simulink model "Compare_lin_nonlin"  (R2019b)
settings: Solver=FixedStepAuto  StartTime=0.0  StopTime=10  FixedStep=0.01  RelTol=1e-3
settings Model: Creator=cambr  LastModifiedBy=cambr

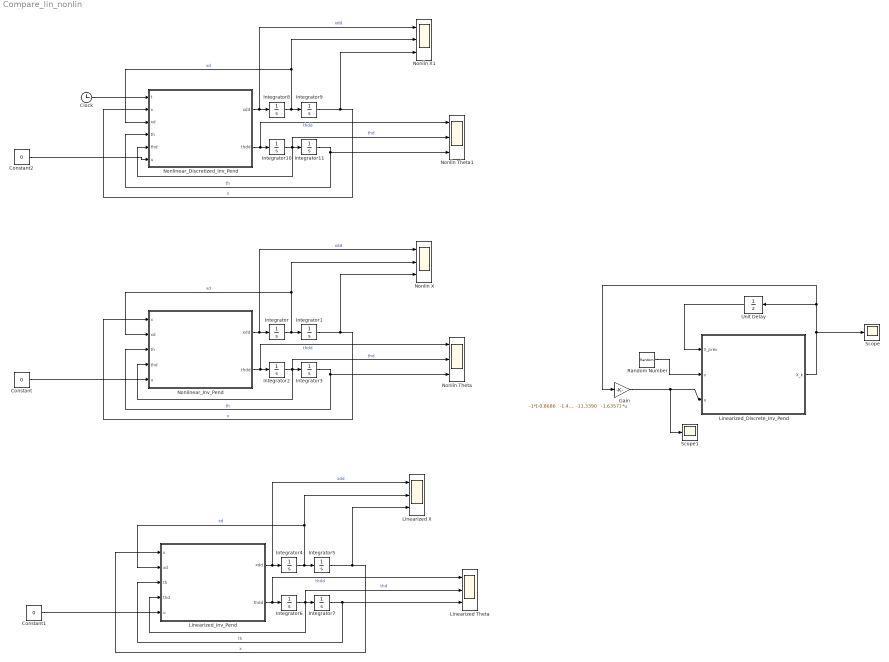
== system Compare_lin_nonlin ==
  Clock : Clock
  Constant : Constant  Value=0
  Constant1 : Constant  Value=0
  Constant2 : Constant  Value=0
  Gain : Gain  Gain="-1*[-0.8686   -1.4350  -11.3390   -1.6357]"  Multiplication=Matrix(K*u)
  Integrator{,1..2,4..6,8..10} (9 alike) : Integrator
  Integrator11 : Integrator  InitialCondition=0.2
  Integrator3 : Integrator  InitialCondition=0.2
  Integrator7 : Integrator  InitialCondition=0.2
  Linearized Theta : Scope  NumInputPorts=3
  Linearized X : Scope  NumInputPorts=3
  Linearized_Discrete_Inv_Pend : MATLAB Function  TreatAsAtomicUnit=on
  Linearized_Inv_Pend : MATLAB Function  TreatAsAtomicUnit=on
  Nonlin Theta : Scope  NumInputPorts=3
  Nonlin Theta1 : Scope  NumInputPorts=3
  Nonlin X : Scope  NumInputPorts=3
  Nonlin X1 : Scope  NumInputPorts=3
  Nonlinear_Discretized_Inv_Pend : MATLAB Function  TreatAsAtomicUnit=on
  Nonlinear_Inv_Pend : MATLAB Function  TreatAsAtomicUnit=on
  Random Number : RandomNumber  Variance=.000001  SampleTime=0.01
  Scope : Scope
  Scope1 : Scope
  Unit Delay : UnitDelay  InitialCondition=[0;0;0.1;0]  SampleTime=-1  HasFrameUpgradeWarning=on
  wires:
  Integrator/1 -> Integrator1/1, Nonlin X/2, Nonlinear_Inv_Pend/2(xd)  "xd"
  Integrator1/1 -> Nonlin X/3, Nonlinear_Inv_Pend/1(x)  "x"
  Nonlinear_Inv_Pend/1(xdd) -> Nonlin X/1, Integrator/1  "xdd"
  Integrator3/1 -> Nonlinear_Inv_Pend/3(th), Nonlin Theta/3  "th"
  Integrator2/1 -> Nonlin Theta/2, Integrator3/1, Nonlinear_Inv_Pend/4(thd)  "thd"
  Nonlinear_Inv_Pend/2(thdd) -> Nonlin Theta/1, Integrator2/1  "thdd"
  Constant/1 -> Nonlinear_Inv_Pend/5(u)
  Integrator5/1 -> Linearized X/3, Linearized_Inv_Pend/1(x)  "x"
  Linearized_Inv_Pend/2(thdd) -> Linearized Theta/1, Integrator6/1  "thdd"
  Constant1/1 -> Linearized_Inv_Pend/5(u)
  Integrator6/1 -> Linearized Theta/2, Integrator7/1, Linearized_Inv_Pend/4(thd)  "thd"
  Integrator7/1 -> Linearized_Inv_Pend/3(th), Linearized Theta/3  "th"
  Linearized_Inv_Pend/1(xdd) -> Linearized X/1, Integrator4/1  "xdd"
  Integrator4/1 -> Integrator5/1, Linearized X/2, Linearized_Inv_Pend/2(xd)  "xd"
  Linearized_Discrete_Inv_Pend/1(X_k) -> Unit Delay/1, Gain/1, Scope/1
  Unit Delay/1 -> Linearized_Discrete_Inv_Pend/1(X_prev)
  Gain/1 -> Linearized_Discrete_Inv_Pend/3(u), Scope1/1
  Random Number/1 -> Linearized_Discrete_Inv_Pend/2(v)
  Constant2/1 -> Nonlinear_Discretized_Inv_Pend/6(u)
  Nonlinear_Discretized_Inv_Pend/1(xdd) -> Nonlin X1/1, Integrator8/1  "xdd"
  Integrator11/1 -> Nonlinear_Discretized_Inv_Pend/4(th), Nonlin Theta1/3  "th"
  Integrator9/1 -> Nonlin X1/3, Nonlinear_Discretized_Inv_Pend/2(x)  "x"
  Integrator10/1 -> Nonlin Theta1/2, Integrator11/1, Nonlinear_Discretized_Inv_Pend/5(thd)  "thd"
  Integrator8/1 -> Integrator9/1, Nonlin X1/2, Nonlinear_Discretized_Inv_Pend/3(xd)  "xd"
  Nonlinear_Discretized_Inv_Pend/2(thdd) -> Nonlin Theta1/1, Integrator10/1  "thdd"
  Clock/1 -> Nonlinear_Discretized_Inv_Pend/1(t)

== matlab function Compare_lin_nonlin/Linearized_Inv_Pend ==
  data: x input size=1; xd input size=1; xdd output size=1; thdd output size=1; th input size=1; thd input size=1; u input
function [xdd, thdd] = fcn(x, xd, th, thd, u)

g = 9.8; % gravity
m = 0.08; % kg, pendulum mass, meas 0.08
M = 0.32; % kg, cart mass, meas 0.32
l = 0.17; % meters, center of mass location on pendulum, meas 0.17
I = 3.5e-3; %1/3*m1*r^2 + m2*L^2;, meas 3.5e-3
b = 0.01; % N/(m/s)

xdd = (u - m*g*th)/(M);
thdd = (u -(M+m)*g*th)/(-M*l);

== matlab function Compare_lin_nonlin/Nonlinear_Inv_Pend ==
  data: x input size=1; xd input size=1; xdd output size=1; thdd output size=1; th input size=1; thd input size=1; u input
function [xdd, thdd] = fcn(x, xd, th, thd, u)

g = 9.8; % gravity
m = 0.08; % kg, pendulum mass, meas 0.08
M = 0.32; % kg, cart mass, meas 0.32
l = 0.17; % meters, center of mass location on pendulum, meas 0.17
I = 3.5e-3; %1/3*m1*r^2 + m2*L^2;, meas 3.5e-3
b = 0.01; % N/(m/s)

xdd = (u + m*l*sin(th)*thd^2 - m*g*cos(th)*sin(th))/(M + m - m*cos(th)^2);
thdd = (u*cos(th) - (M+m)*g*sin(th) + m*l*cos(th)*sin(th)*thd^2)/(m*l*cos(th)^2 - (M+m)*l);

== matlab function Compare_lin_nonlin/Linearized_Discrete_Inv_Pend ==
  data: X_prev input; v input; X_k output; u input
function X_k  = fcn(X_prev,v, u)

Ad = [1.0000    0.0100   -0.0001   -0.0000;
         0    1.0000   -0.0245   -0.0001;
         0         0    1.0036    0.0100;
         0         0    0.7215    1.0036];

Bd = [0.0002;
      0.0313;
      -0.0009;
      -0.1840];
  
Cd = [1     0     0     0;
      0     0     1     0];

  
X_k = Ad*X_prev + Bd*u + [v; 0; v; 0];
%Y_k = Cd*X_k;

== matlab function Compare_lin_nonlin/Nonlinear_Discretized_Inv_Pend ==
  data: t input; x input size=1; xd input size=1; xdd output size=1; thdd output size=1; th input size=1; thd input size=1; u input
function [xdd, thdd] = fcn(t, x, xd, th, thd, u)

Ts = 0.01;
g = 9.8; % gravity
m = 0.08; % kg, pendulum mass, meas 0.08
M = 0.32; % kg, cart mass, meas 0.32
l = 0.17; % meters, center of mass location on pendulum, meas 0.17
I = 3.5e-3; %1/3*m1*r^2 + m2*L^2;, meas 3.5e-3
b = 0.01; % N/(m/s)

%xdd = (u + m*l*sin(th)*thd^2 - m*g*cos(th)*sin(th))/(M + m - m*cos(th)^2);
%thdd = (u*cos(th) - (M+m)*g*sin(th) + m*l*cos(th)*sin(th)*thd^2)/(m*l*cos(th)^2 - (M+m)*l);

x2d =@(x3, x4)((u + m*l*sin(x3)*x4^2 - m*g*cos(x3)*sin(x3))/(M + m - m*cos(x3)^2));
k1x2d = x2d(th, thd);
k2x2d = x2d(th+.5*Ts, thd+.5*k11*Ts);
k3x2d = x2d(th+.5*Ts, thd+.5*k12*Ts);
k4x2d = x2d(th+Ts, thd+k13*Ts);
xdd =  + ((k11+2*k12+2*k13+k14)/6)*Ts; 

x4_dot =@(x3, x4)((u*cos(x3) - (M+m)*g*sin(x3) + m*l*cos(x3)*sin(x3)*x4^2)/(m*l*cos(x3)^2 - (M+m)*l));
